simulink model "chap17_01_03_model"  (R2013b)
settings: Solver=ode3  StartTime=0.0  StopTime=10.0  RelTol=1e-3
settings Model: Creator=sunzx.fnst  LastModifiedBy=sunzx.fnst

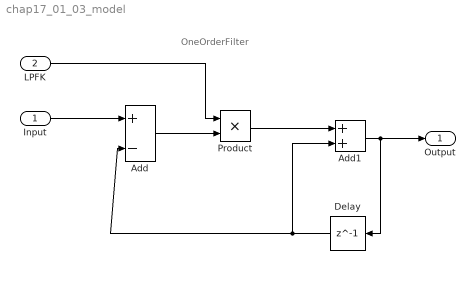
== system chap17_01_03_model ==
  note: OneOrderFilter
  Input : Inport
  LPFK : Inport  Port=2
  Add : Sum  Inputs=+-
  Add1 : Sum
  Delay : Delay  DelayLength=1  InitialCondition=0
  Product : Product
  Output : Outport
  wires:
  Input/1 -> Add/1
  LPFK/1 -> Product/1
  Add/1 -> Product/2
  Product/1 -> Add1/1
  Delay/1 -> Add/2, Add1/2
  Add1/1 -> Output/1, Delay/1
